simulink model "gm_whdlOFDMTransmitter_up_con"  (R2022b)
settings: Solver=FixedStepDiscrete  StartTime=0.0  StopTime=stopTime  RelTol=1e-3
PreLoadFcn:
  | addpath('D:\NU\OF\WHDLOFDMTransmitterExample_all_new\hdl_prj\hdlsrc3\whdlOFDMTransmitter_up_con');
InitFcn:
  | % Initialization
  | whdlexamples.OFDMTransmitterInit;
undefined symbols (not defined in the file or in its folder): compFilt, dataBits, delay, fs, hbFilt, lowpassFilt, outputFrame, TIF
libraries: dsphdlfiltering2 x4, dspsrcs4 x3, hdlsllib x1, dsphdlsigops2 x1, dspsigops x1
CloseFcn:
  | addpath('D:\NU\OF\WHDLOFDMTransmitterExample_all_new\hdl_prj\hdlsrc3\whdlOFDMTransmitter_up_con');
  | rmpath('D:\NU\OF\WHDLOFDMTransmitterExample_all_new\hdl_prj\hdlsrc3\whdlOFDMTransmitter_up_con');
settings Model: Creator=The MathWorks, Inc.  LastModifiedBy=LEGION
settings SolverCC: AlgebraicLoopSolver=TrustRegion
settings DataIOCC: SaveTime=off  ReturnWorkspaceOutputs=off
settings OptimizationCC: BlockReduction=off  ConditionallyExecuteInputs=off  DefaultParameterBehavior=Inlined
settings DebuggingCC: AlgebraicLoopMsg=error  InheritedTsInSrcMsg=none  SingleTaskRateTransMsg=error  UnconnectedInputMsg=warning  UnconnectedOutputMsg=warning  UnconnectedLineMsg=warning  SFMachineParentedDataDiag=warning
settings HardwareCC: ProdBitPerPointer=32  ProdBitPerSizeT=32  ProdBitPerPtrDiffT=32  ProdLargestAtomicFloat=None  ProdIntDivRoundTo=Undefined  ProdEndianess=Unspecified  ProdWordSize=32  ProdHWDeviceType=ASIC/FPGA->ASIC/FPGA  TargetBitPerPointer=64  TargetBitPerSizeT=64  TargetBitPerPtrDiffT=64  TargetLongLongMode=on  TargetIntDivRoundTo=Zero  TargetEndianess=LittleEndian  TargetWordSize=64  TargetHWDeviceType=Custom Processor->MATLAB Host Computer  ProdEqTarget=off
settings ModelReferenceCC: UpdateModelReferenceTargets=IfOutOfDate  EnableRefExpFcnMdlSchedulingChecks=on
settings RTWCC: DLArmComputeVersion=19.05

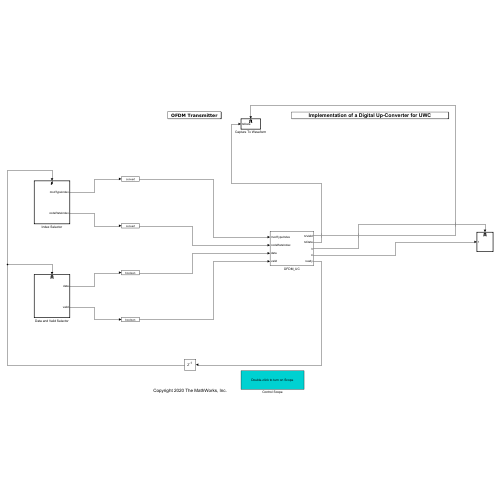
[thumbnail: Simulink's stored preview of the top-level diagram]
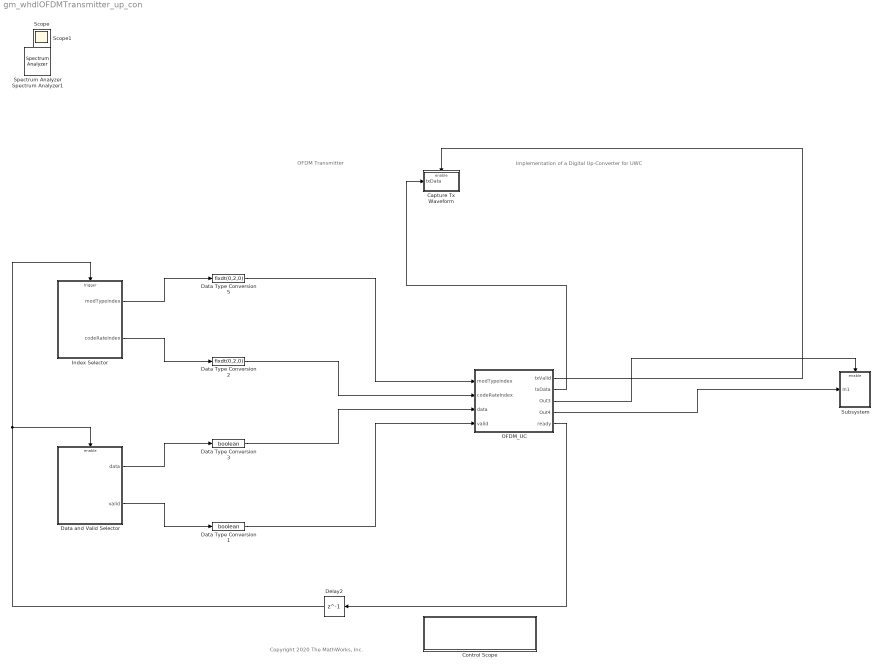
== system gm_whdlOFDMTransmitter_up_con ==
  note: Copyright 2020 The MathWorks, Inc.
  note: OFDM Transmitter
  note: Implementation of a Digital Up-Converter for UWC
  Capture Tx Waveform : Subsystem  TreatAsAtomicUnit=on
  Control Scope : Subsystem
      settings: OpenFcn=|
      | hScopeConfig = get_param([gcs '/Capture Tx Waveform/Spectrum Analyzer'],'ScopeConfiguration');
      | hScopeConfig.Visible = true;
      | clear hScopeConfig;
      mask Display: disp('Double-click to turn on Scope');
  Data Type Conversion1 : DataTypeConversion  OutDataTypeStr=boolean  SaturateOnIntegerOverflow=off  RndMeth=Floor
  Data Type Conversion2 : DataTypeConversion  OutDataTypeStr=fixdt(0,2,0)  RndMeth=Floor
  Data Type Conversion3 : DataTypeConversion  OutDataTypeStr=boolean  SaturateOnIntegerOverflow=off  RndMeth=Floor
  Data Type Conversion5 : DataTypeConversion  OutDataTypeStr=fixdt(0,2,0)  RndMeth=Floor
  Data and Valid Selector : Subsystem  TreatAsAtomicUnit=on
  Delay2 : Delay  DelayLength=1
  Index Selector : Subsystem  TreatAsAtomicUnit=on
  OFDM_UC : Subsystem
  Subsystem : Subsystem
  Scope : Scope
  Scope1 : Scope
  Spectrum Analyzer : SpectrumAnalyzer  IOType=viewer
  Spectrum Analyzer1 : SpectrumAnalyzer  IOType=viewer
  wires:
  Index Selector/1(modTypeIndex) -> Data Type Conversion5/1
  Index Selector/2(codeRateIndex) -> Data Type Conversion2/1
  Delay2/1 -> Index Selector/Trigger, Data and Valid Selector/Enable
  Data and Valid Selector/1(data) -> Data Type Conversion3/1
  Data and Valid Selector/2(valid) -> Data Type Conversion1/1
  Data Type Conversion5/1 -> OFDM_UC/1(modTypeIndex)
  Data Type Conversion2/1 -> OFDM_UC/2(codeRateIndex)
  Data Type Conversion3/1 -> OFDM_UC/3(data)
  Data Type Conversion1/1 -> OFDM_UC/4(valid)
  OFDM_UC/1(txValid) -> Capture Tx Waveform/Enable
  OFDM_UC/2(txData) -> Capture Tx Waveform/1(txData)
  OFDM_UC/3(Out3) -> Subsystem/Enable
  OFDM_UC/4(Out4) -> Subsystem/1(In1)
  OFDM_UC/5(ready) -> Delay2/1

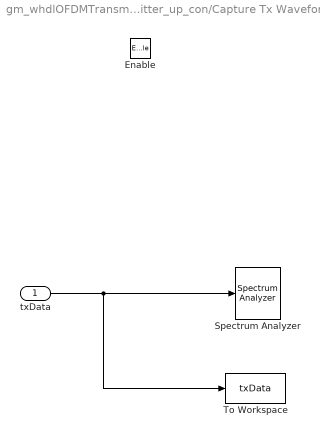
== system gm_whdlOFDMTransmitter_up_con/Capture Tx Waveform ==
  txData : Inport
  Enable : EnablePort
  Spectrum Analyzer : SpectrumAnalyzer
  To Workspace : ToWorkspace  VariableName=txData  SaveFormat=Timeseries  SampleTime=-1
      settings: Save2DSignal=2-D array (concatenate along first dimension)
  wires:
  txData/1 -> Spectrum Analyzer/1, To Workspace/1

== system gm_whdlOFDMTransmitter_up_con/Control Scope ==

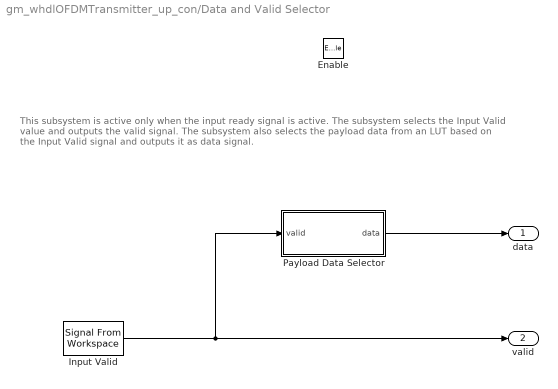
== system gm_whdlOFDMTransmitter_up_con/Data and Valid Selector ==
  note: This subsystem is active only when the input ready signal is active. The subsystem selects the Input Valid value and outputs the valid signal.
      | The subsystem also selects the payload data from an LUT based on the Input Valid signal and outputs it as data signal.
  Enable : EnablePort
  Input Valid : dspsrcs4/Signal From Workspace  X=validIn  Ts=1/(fs*16)  nsamps=1  OutputAfterFinalValue=Setting to zero  ignoreOrWarnInputAndFrameLengths=off  OutputFrames=off
  Payload Data Selector : Subsystem  TreatAsAtomicUnit=on
  data : Outport  InitialOutput=0  VectorParamsAs1DForOutWhenUnconnected=off
  valid : Outport  Port=2  InitialOutput=0  VectorParamsAs1DForOutWhenUnconnected=off
  wires:
  Input Valid/1 -> Payload Data Selector/1(valid), valid/1
  Payload Data Selector/1(data) -> data/1

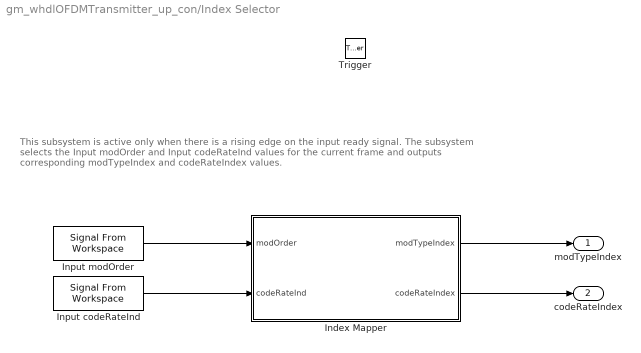
== system gm_whdlOFDMTransmitter_up_con/Index Selector ==
  note: This subsystem is active only when there is a rising edge on the input ready signal. The subsystem selects the Input modOrder and Input codeRateInd values
      | for the current frame and outputs corresponding modTypeIndex and codeRateIndex values.
  Trigger : TriggerPort  VariantControl=(inherit)  PortDimensions=1
  Index Mapper : MATLAB Function  TreatAsAtomicUnit=on
  Input codeRateInd : dspsrcs4/Signal From Workspace  X=codeRateIndex  Ts=-1  nsamps=1  OutputAfterFinalValue=Setting to zero  ignoreOrWarnInputAndFrameLengths=off  OutputFrames=off
  Input modOrder : dspsrcs4/Signal From Workspace  X=modOrder  Ts=-1  nsamps=1  OutputAfterFinalValue=Setting to zero  ignoreOrWarnInputAndFrameLengths=off  OutputFrames=off
  modTypeIndex : Outport  InitialOutput=0  VectorParamsAs1DForOutWhenUnconnected=off
  codeRateIndex : Outport  Port=2  InitialOutput=0  VectorParamsAs1DForOutWhenUnconnected=off
  wires:
  Index Mapper/1(modTypeIndex) -> modTypeIndex/1
  Index Mapper/2(codeRateIndex) -> codeRateIndex/1
  Input modOrder/1 -> Index Mapper/1(modOrder)
  Input codeRateInd/1 -> Index Mapper/2(codeRateInd)

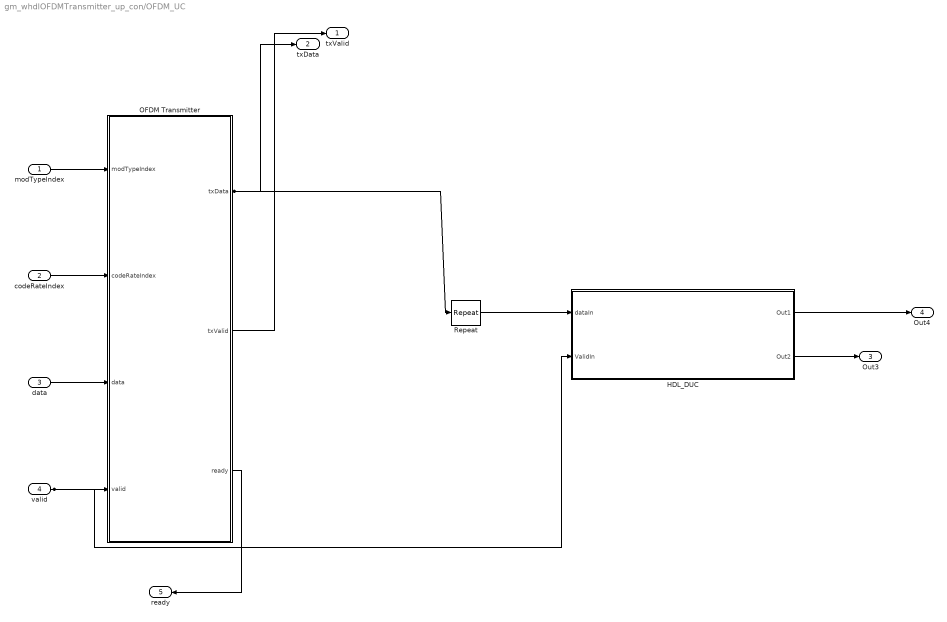
== system gm_whdlOFDMTransmitter_up_con/OFDM_UC ==
  modTypeIndex : Inport
  codeRateIndex : Inport  Port=2
  data : Inport  Port=3
  valid : Inport  Port=4
  HDL_DUC : Subsystem
  OFDM Transmitter : Subsystem
  Repeat : dspsigops/Repeat  N=16  InputProcessing=Columns as channels (frame based)  RateOptions=Allow multirate processing  ic=0  mode=Unused parameter value
  txValid : Outport
  txData : Outport  Port=2
  Out3 : Outport  Port=3
  Out4 : Outport  Port=4
  ready : Outport  Port=5
  wires:
  Repeat/1 -> HDL_DUC/1(dataIn)
  HDL_DUC/2(Out2) -> Out3/1
  HDL_DUC/1(Out1) -> Out4/1
  OFDM Transmitter/3(ready) -> ready/1
  codeRateIndex/1 -> OFDM Transmitter/2(codeRateIndex)
  valid/1 -> OFDM Transmitter/4(valid), HDL_DUC/2(ValidIn)
  data/1 -> OFDM Transmitter/3(data)
  modTypeIndex/1 -> OFDM Transmitter/1(modTypeIndex)
  OFDM Transmitter/2(txValid) -> txValid/1
  OFDM Transmitter/1(txData) -> Repeat/1, txData/1

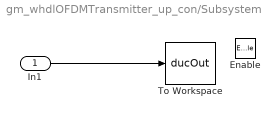
== system gm_whdlOFDMTransmitter_up_con/Subsystem ==
  In1 : Inport
  Enable : EnablePort
  To Workspace : ToWorkspace  VariableName=ducOut  SampleTime=-1
      settings: Save2DSignal=2-D array (concatenate along first dimension)
  wires:
  In1/1 -> To Workspace/1

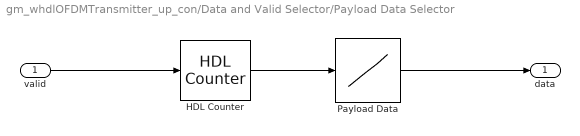
== system gm_whdlOFDMTransmitter_up_con/Data and Valid Selector/Payload Data Selector ==
  valid : Inport
  HDL Counter : hdlsllib/Sources/HDL Counter  CountType=Count limited  CountInit=0  CountStep=1  CountMax=length(dataBits) -1  CountFromType=Initial value  CountFrom=0  CountResetPort=off  CountLoadPort=off  CountEnbPort=on  CountDirPort=off  CountHitOutputPort=off  CountDataType=Unsigned  CountWordLen=nextpow2(length(dataBits))  CountFracLen=0  CountSampTime=1
  Payload Data : Lookup_n-D  NumberOfTableDimensions=1  LookupTableObject=''  BreakpointsForDimension1=0:(length(dataBits) -1)  BreakpointsForDimension1FirstPoint=10  BreakpointsForDimension2FirstPoint=10  BreakpointsForDimension1Spacing=12  BreakpointsForDimension2Spacing=12  IndexSearchMethod=Evenly spaced points  Table=dataBits  InterpMethod=Flat  DiagnosticForOutOfRangeInput=Error  InternalRulePriority=Speed  OutDataTypeStr=fixdt(0,1,0)  RndMeth=Simplest
  data : Outport  InitialOutput=0  VectorParamsAs1DForOutWhenUnconnected=off
  wires:
  HDL Counter/1 -> Payload Data/1
  Payload Data/1 -> data/1
  valid/1 -> HDL Counter/1

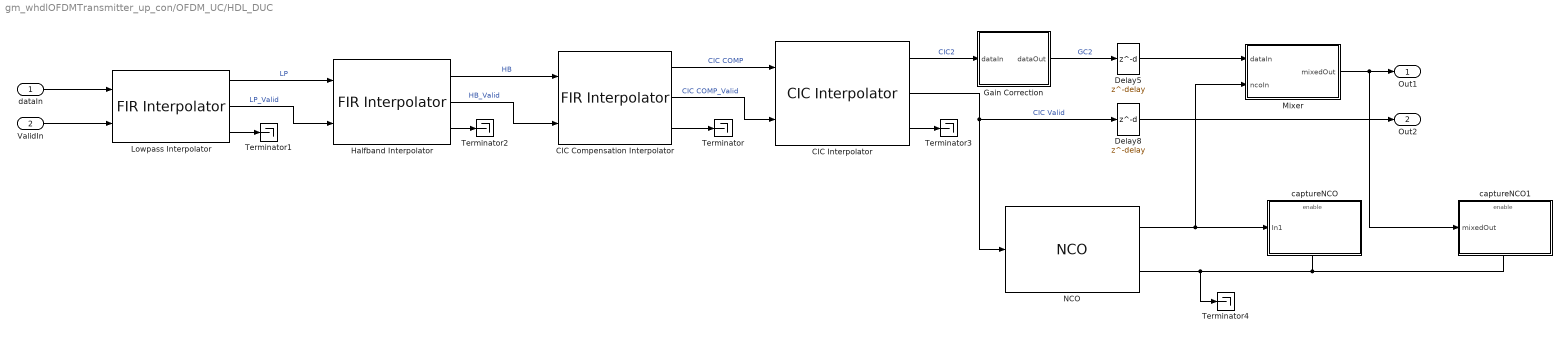
== system gm_whdlOFDMTransmitter_up_con/OFDM_UC/HDL_DUC ==
  dataIn : Inport
  ValidIn : Inport  Port=2
  CIC Compensation Interpolator : dsphdlfiltering2/FIR Interpolator  Numerator=compFilt.Numerator  FilterStructure=Direct form systolic  InterpolationFactor=compFilt.InterpolationFactor  NumCycles=ceil(TIF/(lowpassFilt.InterpolationFactor*hbFilt.InterpolationFactor*outputFrame))  SimulateUsing=Code generation  roundingMode=Floor  overflowMode=off  CoefficientsDataTypeStr=Inherit: Same word length as input  OutputDataTypeStr=fixdt(1,18,14)  ResetInputPort=off  HDLGlobalReset=off
  CIC Interpolator : dsphdlfiltering2/CIC Interpolator  InterpolationSource=Property  InterpolationFactor=cicFilt.InterpolationFactor  MaxInterpolationFactor=8  DifferentialDelay=1  NumSections=3  NumCycles=ceil(TIF/(lowpassFilt.InterpolationFactor*hbFilt.InterpolationFactor*compFilt.InterpolationFactor*outputFrame))  GainCorrection=off  SimulateUsing=Code generation  OutputDataType=Minimum section word lengths  OutputWordLength=18  ResetInputPort=off  HDLGlobalReset=off
  Delay5 : Delay  DelayLength=delay  InitialCondition=0
  Delay8 : Delay  DelayLength=delay  InitialCondition=0
  Gain Correction : Subsystem
  Halfband Interpolator : dsphdlfiltering2/FIR Interpolator  Numerator=hbFilt.Numerator  FilterStructure=Direct form systolic  InterpolationFactor=hbFilt.InterpolationFactor  NumCycles=ceil(TIF/(lowpassFilt.InterpolationFactor*outputFrame))  SimulateUsing=Code generation  roundingMode=Floor  overflowMode=off  CoefficientsDataTypeStr=Inherit: Same word length as input  OutputDataTypeStr=fixdt(1,18,14)  ResetInputPort=off  HDLGlobalReset=off
  Lowpass Interpolator : dsphdlfiltering2/FIR Interpolator  Numerator=lowpassFilt.Numerator  FilterStructure=Direct form systolic  InterpolationFactor=lowpassFilt.InterpolationFactor  NumCycles=ceil(TIF/outputFrame)  SimulateUsing=Code generation  roundingMode=Floor  overflowMode=off  CoefficientsDataTypeStr=Inherit: Same word length as input  OutputDataTypeStr=fixdt(1,18,14)  ResetInputPort=off  HDLGlobalReset=off
  Mixer : Subsystem
  NCO : dsphdlsigops2/NCO  PhaseIncrementSource=Property  PhaseIncrement=nco.PhaseInc  PhaseOffsetSource=Property  PhaseOffset=0  DitherSource=Property  NumDitherBits=nco.NumDitherBits  SamplesPerFrame=outputFrame  LUTCompress=on  ResetAction=off  Waveform=Complex exponential  PhasePort=off  SimulateUsing=Code generation  AccumulatorWL=nco.AccWL  PhaseQuantization=on  NumQuantizerAccumulatorBits=nco.QuantAccWL  OutputDataType=Binary point scaling  OutputWL=18  OutputFL=16
  Terminator{,1..4} (5 alike) : Terminator
  captureNCO : Subsystem
  captureNCO1 : Subsystem
  Out1 : Outport
  Out2 : Outport  Port=2
  wires:
  Lowpass Interpolator/1 -> Halfband Interpolator/1  "LP"
  Lowpass Interpolator/2 -> Halfband Interpolator/2  "LP_Valid"
  Halfband Interpolator/1 -> CIC Compensation Interpolator/1  "HB"
  Halfband Interpolator/2 -> CIC Compensation Interpolator/2  "HB_Valid"
  CIC Compensation Interpolator/1 -> CIC Interpolator/1  "CIC COMP"
  CIC Compensation Interpolator/2 -> CIC Interpolator/2  "CIC COMP_Valid"
  CIC Interpolator/2 -> NCO/1, Delay8/1  "CIC Valid"
  CIC Interpolator/1 -> Gain Correction/1(dataIn)  "CIC2"
  Gain Correction/1(dataOut) -> Delay5/1  "GC2"
  Delay8/1 -> Out2/1
  NCO/1 -> Mixer/2(ncoIn), captureNCO/1(In1)
  NCO/2 -> Terminator4/1, captureNCO1/Enable, captureNCO/Enable
  Delay5/1 -> Mixer/1(dataIn)
  Mixer/1(mixedOut) -> captureNCO1/1(mixedOut), Out1/1
  CIC Compensation Interpolator/3 -> Terminator/1
  Halfband Interpolator/3 -> Terminator2/1
  Lowpass Interpolator/3 -> Terminator1/1
  ValidIn/1 -> Lowpass Interpolator/2
  CIC Interpolator/3 -> Terminator3/1
  dataIn/1 -> Lowpass Interpolator/1

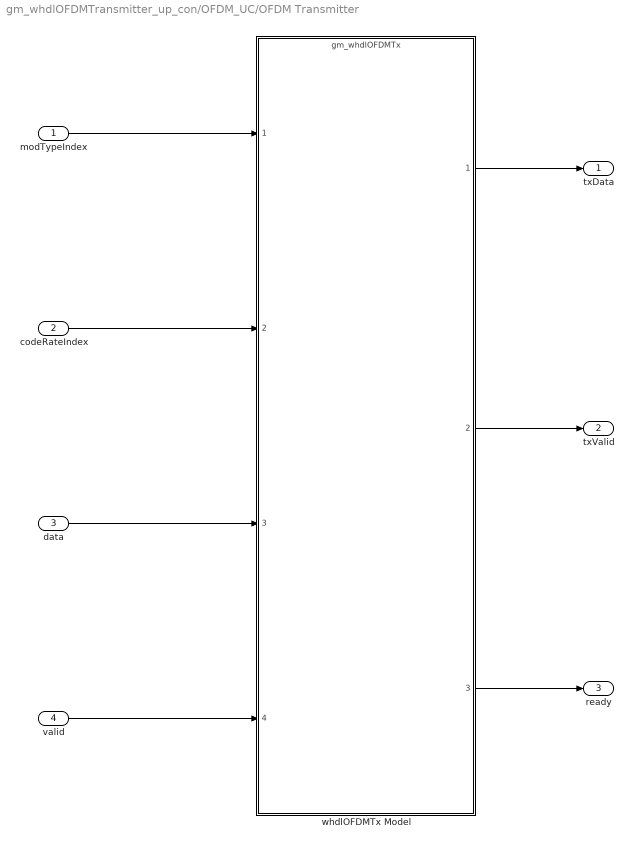
== system gm_whdlOFDMTransmitter_up_con/OFDM_UC/OFDM Transmitter ==
  modTypeIndex : Inport  OutDataTypeStr=fixdt(0, 2, 0)  PortDimensions=1  SampleTime=4.8828125e-07
  codeRateIndex : Inport  Port=2  OutDataTypeStr=fixdt(0, 2, 0)  PortDimensions=1  SampleTime=4.8828125e-07
  data : Inport  Port=3  OutDataTypeStr=boolean  PortDimensions=1  SampleTime=4.8828125e-07
  valid : Inport  Port=4  OutDataTypeStr=boolean  PortDimensions=1  SampleTime=4.8828125e-07
  whdlOFDMTx Model : ModelReference  ModelNameDialog=gm_whdlOFDMTx  ModelReferenceVersion=4.9
  txData : Outport  SampleTime=7.8125e-06  VectorParamsAs1DForOutWhenUnconnected=off
  txValid : Outport  Port=2  SampleTime=7.8125e-06  VectorParamsAs1DForOutWhenUnconnected=off
  ready : Outport  Port=3  SampleTime=4.8828125e-07  VectorParamsAs1DForOutWhenUnconnected=off
  wires:
  modTypeIndex/1 -> whdlOFDMTx Model/1
  codeRateIndex/1 -> whdlOFDMTx Model/2
  data/1 -> whdlOFDMTx Model/3
  valid/1 -> whdlOFDMTx Model/4
  whdlOFDMTx Model/1 -> txData/1
  whdlOFDMTx Model/2 -> txValid/1
  whdlOFDMTx Model/3 -> ready/1

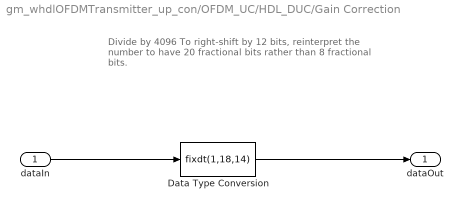
== system gm_whdlOFDMTransmitter_up_con/OFDM_UC/HDL_DUC/Gain Correction ==
  note: Divide by 4096
      | To right-shift by 12 bits, reinterpret the number to have
      | 20 fractional bits rather than 8 fractional bits.
  dataIn : Inport
  Data Type Conversion : DataTypeConversion  OutDataTypeStr=fixdt(1,18,14)  ConvertRealWorld=Stored Integer (SI)  SaturateOnIntegerOverflow=off  RndMeth=Floor
  dataOut : Outport  VectorParamsAs1DForOutWhenUnconnected=off
  wires:
  dataIn/1 -> Data Type Conversion/1
  Data Type Conversion/1 -> dataOut/1

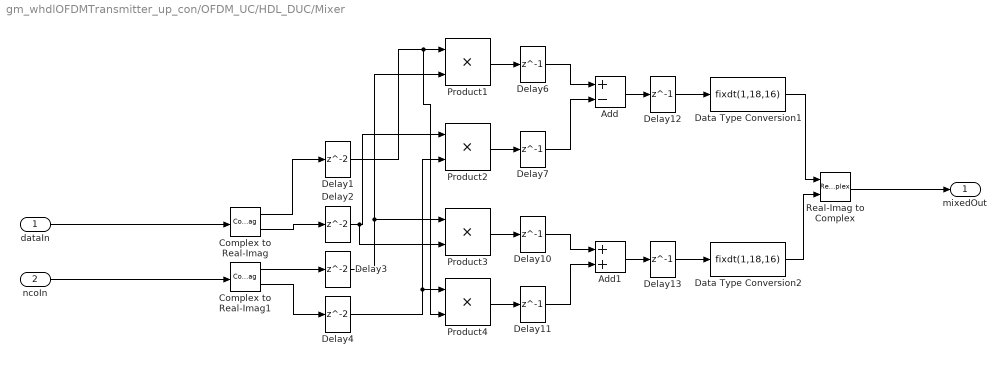
== system gm_whdlOFDMTransmitter_up_con/OFDM_UC/HDL_DUC/Mixer ==
  dataIn : Inport
  ncoIn : Inport  Port=2
  Add : Sum  Inputs=+-
  Add1 : Sum
  Complex to Real-Imag : ComplexToRealImag
  Complex to Real-Imag1 : ComplexToRealImag
  Data Type Conversion1 : DataTypeConversion  OutDataTypeStr=fixdt(1,18,16)  SaturateOnIntegerOverflow=off  RndMeth=Floor
  Data Type Conversion2 : DataTypeConversion  OutDataTypeStr=fixdt(1,18,16)  SaturateOnIntegerOverflow=off  RndMeth=Floor
  Delay{1..4} (4 alike) : Delay  InitialCondition=0
  Delay{6..7,10..13} (6 alike) : Delay  DelayLength=1  InitialCondition=0
  Product{1..4} (4 alike) : Product
  Real-Imag to Complex : RealImagToComplex
  mixedOut : Outport
  wires:
  Delay10/1 -> Add1/1
  Delay11/1 -> Add1/2
  Delay1/1 -> Product1/1, Product4/2
  ncoIn/1 -> Complex to Real-Imag1/1
  Product1/1 -> Delay6/1
  Product2/1 -> Delay7/1
  Delay7/1 -> Add/2
  Complex to Real-Imag1/2 -> Delay4/1
  Complex to Real-Imag/1 -> Delay1/1
  Data Type Conversion2/1 -> Real-Imag to Complex/2
  Delay6/1 -> Add/1
  Delay13/1 -> Data Type Conversion2/1
  Add/1 -> Delay12/1
  Delay4/1 -> Product2/2, Product4/1
  Delay12/1 -> Data Type Conversion1/1
  Delay2/1 -> Product2/1, Product3/2
  Real-Imag to Complex/1 -> mixedOut/1
  dataIn/1 -> Complex to Real-Imag/1
  Complex to Real-Imag1/1 -> Delay3/1
  Add1/1 -> Delay13/1
  Delay3/1 -> Product1/2, Product3/1
  Complex to Real-Imag/2 -> Delay2/1
  Data Type Conversion1/1 -> Real-Imag to Complex/1
  Product3/1 -> Delay10/1
  Product4/1 -> Delay11/1

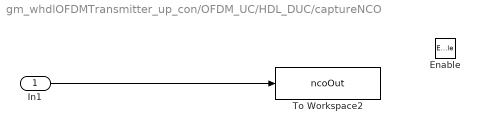
== system gm_whdlOFDMTransmitter_up_con/OFDM_UC/HDL_DUC/captureNCO ==
  In1 : Inport
  Enable : EnablePort
  To Workspace2 : ToWorkspace  VariableName=ncoOut  SampleTime=-1
      settings: Save2DSignal=2-D array (concatenate along first dimension)
  wires:
  In1/1 -> To Workspace2/1

== system gm_whdlOFDMTransmitter_up_con/OFDM_UC/HDL_DUC/captureNCO1 ==
  mixedOut : Inport
  Enable : EnablePort
  To Workspace2 : ToWorkspace  VariableName=ModulatedOut  SampleTime=-1
      settings: Save2DSignal=2-D array (concatenate along first dimension)
  wires:
  mixedOut/1 -> To Workspace2/1

== matlab function gm_whdlOFDMTransmitter_up_con/Index Selector/Index Mapper ==
  data: modOrder input; modTypeIndex output; codeRateInd input; codeRateIndex output
function [modTypeIndex, codeRateIndex] = indexMapper(modOrder, codeRateInd)
%#codegen

    switch modOrder
        case 2                          % BPSK
            modTypeIndex = 0;
        case 4                          % QPSK 
            modTypeIndex = 1;
        case 16                         % 16QAM 
            modTypeIndex = 2;
        case 64                         % 64QAM
            modTypeIndex = 3;
        otherwise
            modTypeIndex = 1;    
    end
    
    switch codeRateInd
        case 0                          % '1/2'
            codeRateIndex = 0;
        case 1                          % '2/3'
            codeRateIndex = 1;
        case 2                          % '3/4'
            codeRateIndex = 2;
        case 3                          % '5/6'
            codeRateIndex = 3;
        otherwise
            codeRateIndex = 0;   
    end
end
